simulink model "Modelo_con_sweep"  (R2020a)
settings: Solver=ode15s  StartTime=0.0  StopTime=140  FixedStep=0.001  MaxStep=0.001  RelTol=1e-3
undefined symbols (not defined in the file): A, Amp, B, ba, Cc, D, f, I_max, K_motor_virtual, ksi, ksia, L, R, R_control, v0, x0
libraries: dspstat3 x1
settings Model: Creator=Noxi-PC  LastModifiedBy=Noxi-PC

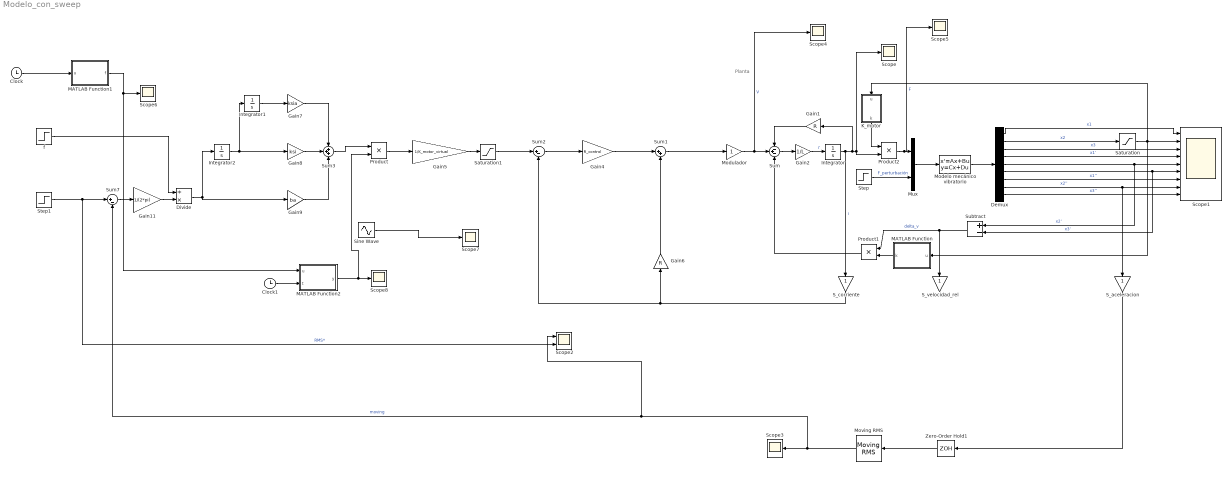
== system Modelo_con_sweep ==
  note: Planta
  Clock : Clock
  Clock1 : Clock
  Demux : Demux  Outputs=9
  Divide : Product  Inputs=/*
  Gain1 : Gain  Gain=R
  Gain11 : Gain  Gain=1/(2*pi)
  Gain2 : Gain  Gain=1/L
  Gain4 : Gain  Gain=R_control
  Gain5 : Gain  Gain=1/K_motor_virtual
  Gain6 : Gain  Gain=R
  Gain7 : Gain  Gain=ksia
  Gain8 : Gain  Gain=ksi
  Gain9 : Gain  Gain=ba
  Integrator : Integrator
  Integrator1 : Integrator
  Integrator2 : Integrator
  K_motor : MATLAB Function  TreatAsAtomicUnit=on
  MATLAB Function : MATLAB Function  TreatAsAtomicUnit=on
  MATLAB Function1 : MATLAB Function  TreatAsAtomicUnit=on
  MATLAB Function2 : MATLAB Function  TreatAsAtomicUnit=on
  Modelo mecánico vibratorio : StateSpace  A=A  B=B  C=Cc  D=D  InitialCondition=[x0,v0]
  Modulador : Gain
  Moving RMS : dspstat3/Moving RMS  Method=Sliding window  ForgettingFactorPort=off  SpecifyWindowLength=on  WindowLength=Ventana  ForgettingFactor=0.99  SimulateUsing=Code generation
      settings: SourceProductBaseCode=DS
  Mux : Mux  Inputs=2
  Product : Product
  Product1 : Product
  Product2 : Product
  S_aceleracion : Gain
  S_corriente : Gain
  S_velocidad_rel : Gain
  Saturation : Saturate  UpperLimit=12.7e-3  LowerLimit=-12.7e-3
  Saturation1 : Saturate  UpperLimit=I_max  LowerLimit=-I_max
  Scope{,3..8} (7 alike) : Scope
  Scope1 : Scope  NumInputPorts=9
  Scope2 : Scope  NumInputPorts=2
  Sine Wave : Sin  Frequency=2*pi*f  SampleTime=0
  Step : Step  Time=3  After=0  SampleTime=0
  Step1 : Step  After=Amp/sqrt(2)  SampleTime=0
  Subtract : Sum  Inputs=+-
  Sum : Sum  Inputs=-+-
  Sum1 : Sum  Inputs=|++
  Sum2 : Sum  Inputs=|+-
  Sum3 : Sum  Inputs=+++
  Sum7 : Sum  Inputs=|+-
  Zero-Order Hold1 : ZeroOrderHold  SampleTime=-1
  f : Step  Time=0  After=f  SampleTime=0
  wires:
  Modelo mecánico vibratorio/1 -> Demux/1
  Demux/1 -> Scope1/1  "x1"
  Demux/2 -> Saturation/1  "x2"
  Demux/3 -> Scope1/3  "x3"
  Demux/4 -> Scope1/4  "x1'"
  Demux/5 -> Scope1/5, Subtract/1  "x2'"
  Demux/6 -> Scope1/6, Subtract/2  "x3'"
  Demux/7 -> Scope1/7  "x1''"
  Demux/8 -> Scope1/8, S_aceleracion/1  "x2''"
  Demux/9 -> Scope1/9  "x3''"
  Mux/1 -> Modelo mecánico vibratorio/1
  Sum/1 -> Gain2/1
  Integrator/1 -> S_corriente/1, Product2/2, Scope/1, Gain1/1  "i"
  Gain1/1 -> Sum/1
  Gain2/1 -> Integrator/1  "i'"
  Step/1 -> Mux/2  "F_perturbación"
  Product1/1 -> Sum/3
  Subtract/1 -> Product1/1, S_velocidad_rel/1  "delta_v"
  Modulador/1 -> Scope4/1, Sum/2  "V"
  Sum2/1 -> Gain4/1
  Gain5/1 -> Saturation1/1
  S_corriente/1 -> Gain6/1, Sum2/2
  Gain4/1 -> Sum1/1
  Gain8/1 -> Sum3/2
  Gain7/1 -> Sum3/1
  Gain9/1 -> Sum3/3
  Integrator1/1 -> Gain7/1
  Integrator2/1 -> Integrator1/1, Gain8/1
  S_aceleracion/1 -> Zero-Order Hold1/1
  Zero-Order Hold1/1 -> Moving RMS/1
  Step1/1 -> Scope2/2, Sum7/1  "RMS*"
  Moving RMS/1 -> Scope2/1, Sum7/2, Scope3/1  "moving"
  Sum7/1 -> Gain11/1
  Sum3/1 -> Product/1
  Saturation/1 -> K_motor/1(u), MATLAB Function/1(u), Scope1/2
  Product2/1 -> Scope5/1, Mux/1  "F"
  K_motor/1(k) -> Product2/1
  MATLAB Function/1(k) -> Product1/2
  Sum1/1 -> Modulador/1
  Divide/1 -> Gain9/1, Integrator2/1
  Gain11/1 -> Divide/2
  Product/1 -> Gain5/1
  Saturation1/1 -> Sum2/1
  Gain6/1 -> Sum1/2
  Clock/1 -> MATLAB Function1/1(u)
  MATLAB Function1/1(f) -> MATLAB Function2/1(u), Scope6/1
  Clock1/1 -> MATLAB Function2/2(t)
  MATLAB Function2/1(y) -> Product/2, Scope8/1
  Sine Wave/1 -> Scope7/1
  f/1 -> Divide/1

== matlab function Modelo_con_sweep/MATLAB Function ==
  data: u input; k output
function k= fcn(u)
coefs = [1.88388325014986e-06,1.21220914940963e-07,-0.000604988778285308,-0.000369001905871298,-0.0433714523559467,-0.0474444922489168,51.4222931299995];

k = coefs(1)*u^6+coefs(2)*u^5+coefs(3)*u^4+coefs(4)*u^3+coefs(5)*u^2+coefs(6)*u^1+coefs(7);

== matlab function Modelo_con_sweep/MATLAB Function1 ==
  data: u input; f output
function f = fcn(u)

f = 100* 2^(2*u/60);

== matlab function Modelo_con_sweep/MATLAB Function2 ==
  data: u input; y output; t input
function y = fcn(u,t)

y = sin(2*pi*u*t);

== matlab function Modelo_con_sweep/K_motor ==
  data: u input; k output
function k = fcn(u)
coefs = [1.88388325014986e-06,1.21220914940963e-07,-0.000604988778285308,-0.000369001905871298,-0.0433714523559467,-0.0474444922489168,51.4222931299995];

k = coefs(1)*u^6+coefs(2)*u^5+coefs(3)*u^4+coefs(4)*u^3+coefs(5)*u^2+coefs(6)*u^1+coefs(7);
